simulink model "relay_MFS"  (R2015a)
settings: Solver=ode3  StartTime=0.0  StopTime=1  FixedStep=0.001  RelTol=1e-3
values from neighbouring files (symbols this model uses):
  f_w = 2*pi    (= 6.28318530718)    [ctr.m]
settings Model: Creator=guima  LastModifiedBy=guima

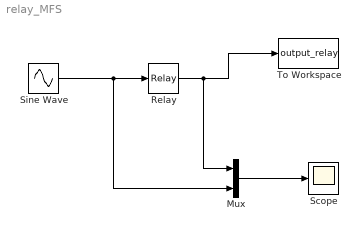
== system relay_MFS ==
  Mux : Mux  Inputs=2
  Relay : Relay  OnOutputValue=2  OffOutputValue=1
  Scope : Scope
  Sine Wave : Sin  Frequency=f_w  SampleTime=0
  To Workspace : ToWorkspace  VariableName=output_relay  SaveFormat=Structure With Time  SampleTime=-1
  wires:
  Mux/1 -> Scope/1
  Relay/1 -> To Workspace/1, Mux/1
  Sine Wave/1 -> Mux/2, Relay/1
